simulink model "angular_position"  (R2022b)
settings: Solver=VariableStepAuto  StartTime=0.0  StopTime=10.0  RelTol=1e-3
libraries: iossensorlib x2
settings Model: PauseTimes=10  Creator=rashmibadri  LastModifiedBy=rashmibadri
settings DebuggingCC: UnconnectedInputMsg=warning  UnconnectedOutputMsg=warning  UnconnectedLineMsg=warning
settings ModelReferenceCC: EnableRefExpFcnMdlSchedulingChecks=on
settings RTWCC: DLArmComputeVersion=19.05

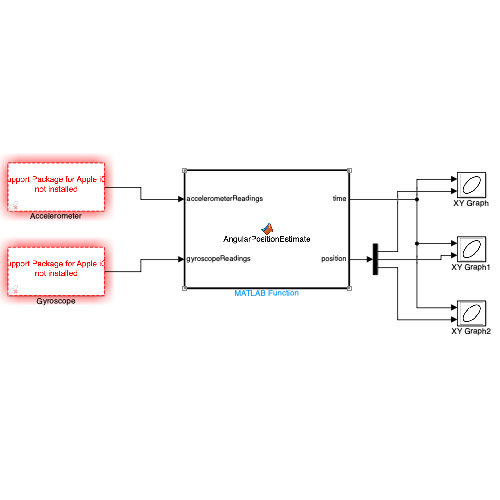
[thumbnail: Simulink's stored preview of the top-level diagram]
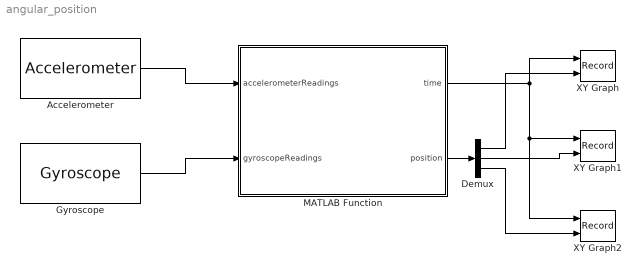
== system angular_position ==
  Accelerometer : iossensorlib/Accelerometer  OutputVector_=on  SampleTime_=0.1  blockPlatform=iOS
  Demux : Demux  Outputs=3
  Gyroscope : iossensorlib/Gyroscope  OutputVector_=on  SampleTime_=0.1  blockPlatform=iOS
  MATLAB Function : MATLAB Function  TreatAsAtomicUnit=on
  XY Graph : Record  FileSettingsInternal="{\"entries\":[{\"content\":{\"excelSettings\":{\"content\":{},\"type\":\"Streamout.ExcelSettings\"}},\"type\":\"Streamout.FileSettingStorage\",\"uuid\":\"eacdf5e5-39c3-46f3-87f7-e198afbab46d\"}],\"packageUris\":[\"http://schema.mathworks.com/mf0/streamout_blocks/R2020a\"],\"version\":\"1.0\"}"  Layout=[1 1]  SignalsInternal="{\"entries\":[{\"content\":{\"signals\":[{\"content\":{\"blockPath\":[\"angular_position/XY Graph\"],\"channel\":[],\"dimensions\":[1],\"domain\":\"angular_position/XY Graph\",\"lineColor\":\"#ff13a6\",\"plots\":[],\"port\":1,\"sid\":[],\"signalID\":81,\"signalName\":\"MATLAB Function:1\"},\"type\":\"RecordBlkView.Signal\",\"uuid\":\"cbc6415d-f3e4-40b9-8a3e-f51b57b8fd62\"},{\"content\":{\"blockPath\":[\"angular_position/XY Graph\"],\"channel\":[],\"dimensions\":[1,1],\"domain\":\"angular_position/XY Graph\",\"lineColor\":\"#fe330a\",\"plots\":[],\"port\":2,\"sid\":[],\"signalID\":84,\"signalName\":\"Demux:1\"},\"type\":\"RecordBlkView.Signal\",\"uuid\":\"cd595ed3-0385-476c-8539-97931016f5a3\"}]},\"type\":\"RecordBlkView.InputSignals\",\"uuid\":\"190a52a7-3d6f-4e6e-8ba4-94d00ec28869\"}],\"packageUris\":[\"http://schema.mathworks.com/mf0/streamout_blocks/R2020a\"],\"version\":\"1.0\"}"  VisualizationBindings="{\"xyplotplugin\":{\"info\":[{\"series\":[],\"subplotID\":1}]}}"  CompatibilityTag=XY
  XY Graph1 : Record  FileSettingsInternal="{\"entries\":[{\"content\":{\"excelSettings\":{\"content\":{},\"type\":\"Streamout.ExcelSettings\"}},\"type\":\"Streamout.FileSettingStorage\",\"uuid\":\"36146f92-bbfe-4847-afc3-473cc5833e0c\"}],\"packageUris\":[\"http://schema.mathworks.com/mf0/streamout_blocks/R2020a\"],\"version\":\"1.0\"}"  Layout=[1 1]  SignalsInternal="{\"entries\":[{\"content\":{\"signals\":[{\"content\":{\"blockPath\":[\"angular_position/XY Graph1\"],\"channel\":[],\"dimensions\":[1],\"domain\":\"angular_position/XY Graph1\",\"lineColor\":\"#ff13a6\",\"plots\":[],\"port\":1,\"sid\":[],\"signalID\":73,\"signalName\":\"MATLAB Function:1\"},\"type\":\"RecordBlkView.Signal\",\"uuid\":\"c031c9cf-69b8-4ec0-a7fb-661aa4623e7c\"},{\"content\":{\"blockPath\":[\"angular_position/XY Graph1\"],\"channel\":[],\"dimensions\":[1,1],\"domain\":\"angular_position/XY Graph1\",\"lineColor\":\"#fe330a\",\"plots\":[],\"port\":2,\"sid\":[],\"signalID\":76,\"signalName\":\"Demux:1\"},\"type\":\"RecordBlkView.Signal\",\"uuid\":\"0f937d15-2b57-4b68-be76-1f6e01c203e2\"}]},\"type\":\"RecordBlkView.InputSignals\",\"uuid\":\"66fad60e-320b-469f-99bf-a029054ddf33\"}],\"packageUris\":[\"http://schema.mathworks.com/mf0/streamout_blocks/R2020a\"],\"version\":\"1.0\"}"  VisualizationBindings="{\"xyplotplugin\":{\"info\":[{\"series\":[],\"subplotID\":1}]}}"  CompatibilityTag=XY
  XY Graph2 : Record  FileSettingsInternal="{\"entries\":[{\"content\":{\"excelSettings\":{\"content\":{},\"type\":\"Streamout.ExcelSettings\"}},\"type\":\"Streamout.FileSettingStorage\",\"uuid\":\"022a2347-c227-428f-919d-b0c5b6e76f39\"}],\"packageUris\":[\"http://schema.mathworks.com/mf0/streamout_blocks/R2020a\"],\"version\":\"1.0\"}"  Layout=[1 1]  SignalsInternal="{\"entries\":[{\"content\":{\"signals\":[{\"content\":{\"blockPath\":[\"angular_position/XY Graph2\"],\"channel\":[],\"dimensions\":[1],\"domain\":\"angular_position/XY Graph2\",\"lineColor\":\"#ff13a6\",\"plots\":[],\"port\":1,\"sid\":[],\"signalID\":89,\"signalName\":\"MATLAB Function:1\"},\"type\":\"RecordBlkView.Signal\",\"uuid\":\"cb201b28-bf30-434d-90f1-b7ffa11dd35f\"},{\"content\":{\"blockPath\":[\"angular_position/XY Graph2\"],\"channel\":[],\"dimensions\":[1,1],\"domain\":\"angular_position/XY Graph2\",\"lineColor\":\"#fe330a\",\"plots\":[],\"port\":2,\"sid\":[],\"signalID\":92,\"signalName\":\"Demux:1\"},\"type\":\"RecordBlkView.Signal\",\"uuid\":\"c6b4de51-a4f4-4c8d-a7ce-879bb45c38f2\"}]},\"type\":\"RecordBlkView.InputSignals\",\"uuid\":\"22032a67-dc65-4fe9-8582-8aa2fb9a1f3c\"}],\"packageUris\":[\"http://schema.mathworks.com/mf0/streamout_blocks/R2020a\"],\"version\":\"1.0\"}"  VisualizationBindings="{\"xyplotplugin\":{\"info\":[{\"series\":[],\"subplotID\":1}]}}"  CompatibilityTag=XY
  wires:
  Accelerometer/1 -> MATLAB Function/1(accelerometerReadings)
  Gyroscope/1 -> MATLAB Function/2(gyroscopeReadings)
  MATLAB Function/1(time) -> XY Graph2/1, XY Graph1/1, XY Graph/1
  MATLAB Function/2(position) -> Demux/1
  Demux/1 -> XY Graph/2
  Demux/3 -> XY Graph2/2
  Demux/2 -> XY Graph1/2

== matlab function angular_position/MATLAB Function ==
  data: accelerometerReadings input; gyroscopeReadings input; time output; position output
function [time, position] = AngularPositionEstimate(accelerometerReadings, gyroscopeReadings)
    ld = load('rpy_9axis.mat');
    Fs = ld.Fs;
    decim = 2;
    accelerometerReadings = ld.sensorData.Acceleration;
    gyroscopeReadings = ld.sensorData.AngularVelocity;
    fuse = imufilter;
    %fuse = imufilter('SampleRate',Fs,'DecimationFactor',decim);
    q = fuse(accelerometerReadings,gyroscopeReadings);
    %time = 3;
    position = (eulerd(q,'ZYX','frame'))';
    %position = position(1,:);
    time = 3
    %time = (0:decim:size(accelerometerReadings,1)-1)/Fs;
    %plot(time,eulerd(q,'ZYX','frame'));
end
